simulink model "humanSubject07_48dof_test"  (R2022a)
settings: Solver=VariableStepAuto  StartTime=0.0  StopTime=4.5  RelTol=1e-3
values from neighbouring files (symbols this model uses):
  m = size(marker.links, 1)    [master_thesis_script.m]    (also in trial.m)
  marker = msg.ChildFrameId(14)    [callback_class.m]
  noise =     [noise_S1_F1_H2.mat]    (also in show_Results.m = noise.noise)
  s = s + 1    (= 2)    [Phi_J_generation.m]    (also in master_thesis_script.m; trial.m)
undefined symbols (not defined in the file or in its folder): arm, LS, X, Y, Z
libraries: nesl_utility x105, sm_lib x84
(part 3 of 3)

== system humanSubject07_48dof_test/Human arm/Wrist_joint/Wy_Wz ==
  jRightShoulder_roty_AxisInvTransform : sm_lib/Frames and Transforms/Rigid Transform  TranslationMethod=Cartesian  TranslationStandardOffset=0  TranslationLengthUnit=m  TranslationStandardAxis=+Z  TranslationCartesianOffset=[0, 0, 0]  TranslationROffset=0  TranslationROffsetUnits=m  TranslationZOffset=0  TranslationZOffsetUnits=m  TranslationThetaOffset=0  TranslationThetaOffsetUnits=deg  RotationMethod=ArbitraryAxis  RotationAngleUnits=rad  RotationStandardAxis=+Z  RotationAngle=pi/2  RotationArbitraryAxis=[0, 1, 0]  FollAlignAxisA=+X  BaseAlignAxisA=+Y  FollAlignAxisB=+Y  BaseAlignAxisB=+Z  RotationSequenceAxes=FollowerAxes  RotationSequence=XYX  RotationSequenceAngles=[0 0 0]  RotationSequenceAnglesUnits=deg  RotationMatrix=[1 0 0; 0 1 0; 0 0 1]
  jRightShoulder_roty_AxisInvTransform1 : sm_lib/Frames and Transforms/Rigid Transform  TranslationMethod=Cartesian  TranslationStandardOffset=0  TranslationLengthUnit=m  TranslationStandardAxis=+Z  TranslationCartesianOffset=[0, 0, 0]  TranslationROffset=0  TranslationROffsetUnits=m  TranslationZOffset=0  TranslationZOffsetUnits=m  TranslationThetaOffset=0  TranslationThetaOffsetUnits=deg  RotationMethod=ArbitraryAxis  RotationAngleUnits=rad  RotationStandardAxis=+Z  RotationAngle=pi/2  RotationArbitraryAxis=[0, 0, 1]  FollAlignAxisA=+X  BaseAlignAxisA=+Y  FollAlignAxisB=+Y  BaseAlignAxisB=+Z  RotationSequenceAxes=FollowerAxes  RotationSequence=XYX  RotationSequenceAngles=[0 0 0]  RotationSequenceAnglesUnits=deg  RotationMatrix=[1 0 0; 0 1 0; 0 0 1]
  Wy : PMIOPort  Side=Left
  Wz : PMIOPort  Port=2  Side=Right
  connections:
  Wz/RConn1 -- jRightShoulder_roty_AxisInvTransform1/RConn1
  Wy/RConn1 -- jRightShoulder_roty_AxisInvTransform/LConn1
  jRightShoulder_roty_AxisInvTransform/RConn1 -- jRightShoulder_roty_AxisInvTransform1/LConn1

== matlab function humanSubject07_48dof_test/LS ==
  data: markers input; qdot_LS output [3..100]; markers_link input; pdot_meas input; q_LS input; arm parameter
function qdot_LS = LS(markers, markers_link, pdot_meas, q_LS, arm)
 
% Computes the joints' velocities using a Least Squares approach 

% Inputs:
% -- markers      : matrix containing markers position wrt Base RF of link where they are placed
% -- markers_link : vector containing link {1, 2, 3} depending on where the markers are placed
% -- pdot_meas    : vector containing the markers' velocities in x, y, z
% -- q_LS         : current joint variables configuration

% Output:
% -- qdot_LS      : estimated joints' velocities

% Number of markers
m = height(markers);
% Number of dof (joints)
n = length(q_current);
% Initialization
jacobian_current = zeros(3*m,n);

for i = 1 : m

    [~, jacobian_current(3*(i-1)+1:3*(i-1)+3, :)] = FK_Jacobian_i(markers(i, :), markers_link(i), q_LS, arm);
end 

qdot_LS = eye(7,7) / (jacobian_current' * jacobian_current) * jacobian_current' * pdot_meas;

== matlab function humanSubject07_48dof_test/FK_Jacobian ==
  data: markers input; markers_pos output [3..100]; markers_link input; q input; arm parameter; jacobian output
function [markers_pos, jacobian] = FK_Jacobian_all(markers, markers_link, q, arm)
 
% Computes the markers' positions and velocities

% Inputs:
% -- markers      : matrix containing markers position wrt Base RF of link where they are placed
% -- markers_link : vector containing link {1, 2, 3} depending on where the markers are placed
% -- q            : current joint variables configuration
% -- arm          : arm parameters used to compute the forward kinematics

% Output:
% -- markers_pos    : matrix containing markers position wrt World RF

% Number of markers
m = height(markers);
% Number of dof (joints)
n = length(q);
% Initialization
markers_pos = zeros(m, 3);
jacobian = zeros(3*m,n);

% Compute markers position and jacobian evaluated at q
for i = 1 : m

    [markers_pos(i, :), jacobian(3*(i-1)+1:3*(i-1)+3, :)] = FK_Jacobian_i(markers(i, :), markers_link(i), q, arm);
end
